simulink model "lab2clrun"  (Simulink 8.9)
settings: Solver=ode45  StartTime=0.0  StopTime=10  RelTol=1e-3  EnableMultiTasking=on
libraries: simulink_extras x1
settings Model: Creator=Mark  LastModifiedBy=ngriffith
settings OptimizationCC: ExpressionDepthLimit=2147483647  InitFltsAndDblsToZero=on
settings DebuggingCC: SaveWithParameterizedLinksMsg=none  SignalResolutionControl=TryResolveAllWithWarning  SolverPrmCheckMsg=warning  MultiTaskDSMMsg=warning  MultiTaskCondExecSysMsg=none
settings GRTTargetCC: TargetFcnLib=ansi_tfl_tmw.mat

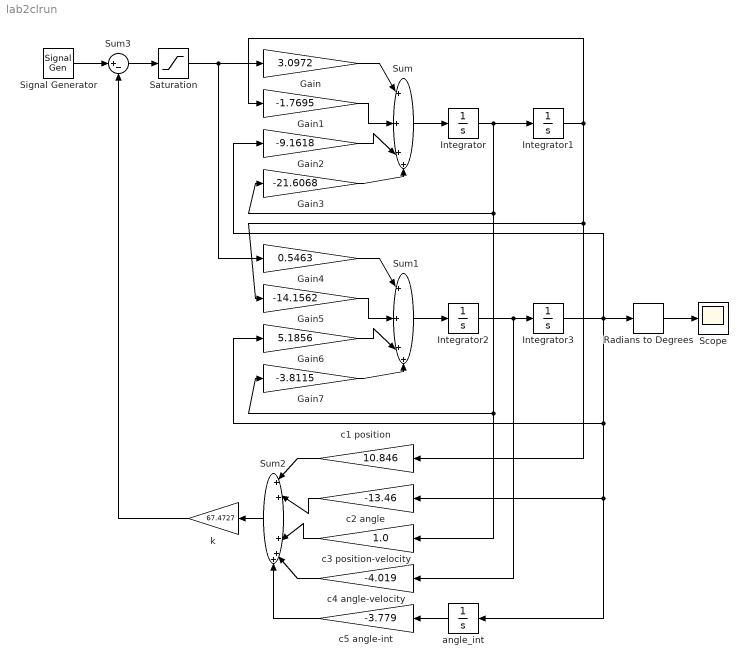
== system lab2clrun ==
  Gain : Gain  Gain=3.0972
  Gain1 : Gain  Gain=-1.7695
  Gain2 : Gain  Gain=-9.1618
  Gain3 : Gain  Gain=-21.6068
  Gain4 : Gain  Gain=0.5463
  Gain5 : Gain  Gain=-14.1562
  Gain6 : Gain  Gain=5.1856
  Gain7 : Gain  Gain=-3.8115
  Integrator{,1..3} (4 alike) : Integrator
  Radians to Degrees : simulink_extras/Transformations/Radians to Degrees
  Saturation : Saturate  UpperLimit=22  LowerLimit=-22
  Scope : Scope
  Signal Generator : SignalGenerator  WaveForm=random  Amplitude=2  Frequency=0.1
  Sum : Sum  Inputs=|++++
  Sum1 : Sum  Inputs=|++++
  Sum2 : Sum  Inputs=|++|+++
  Sum3 : Sum  Inputs=|+-
  angle_int : Integrator
  c1 position : Gain  Gain=10.846
  c2 angle : Gain  Gain=-13.46
  c3 position-velocity : Gain  Gain=1.0
  c4 angle-velocity : Gain  Gain=-4.019
  c5 angle-int : Gain  Gain=-3.779
  k : Gain  Gain=67.4727
  wires:
  Gain3/1 -> Sum/4
  Gain1/1 -> Sum/2
  Gain/1 -> Sum/1
  Sum/1 -> Integrator/1
  Integrator/1 -> Integrator1/1, Gain3/1, Gain7/1, c3 position-velocity/1
  Gain7/1 -> Sum1/4
  Gain6/1 -> Sum1/3
  Gain5/1 -> Sum1/2
  Gain4/1 -> Sum1/1
  Sum1/1 -> Integrator2/1
  Integrator2/1 -> Integrator3/1, c4 angle-velocity/1
  c3 position-velocity/1 -> Sum2/3
  c2 angle/1 -> Sum2/2
  c1 position/1 -> Sum2/1
  c5 angle-int/1 -> Sum2/5
  c4 angle-velocity/1 -> Sum2/4
  Sum2/1 -> k/1
  Sum3/1 -> Saturation/1
  k/1 -> Sum3/2
  angle_int/1 -> c5 angle-int/1
  Signal Generator/1 -> Sum3/1
  Saturation/1 -> Gain/1, Gain4/1
  Integrator1/1 -> Gain1/1, Gain5/1, c1 position/1
  Integrator3/1 -> Radians to Degrees/1, Gain6/1, c2 angle/1, angle_int/1, Gain2/1
  Gain2/1 -> Sum/3
  Radians to Degrees/1 -> Scope/1
